simulink model "Back2BackSim1"  (R2017a)
settings: Solver=VariableStepAuto  StartTime=0.0  StopTime=.2  RelTol=1e-3
undefined symbols (not defined in the file or in its folder): st_time3
libraries: fl_lib x62, nesl_utility x32, powerlib_meascontrol x8, powerlib x1, elec_lib x1
(part 2 of 2)

== matlab function Back2BackSim1/PowerControlLoop_4CSI/Instantaneous p-q transformation ==
  data: va input; p output; vb input; vc input; ia input; ib input; ic input; q output; p0 output; iac output; ibc output; icc output; ialphC output; ibetaC output; ValA output; VbetA output
function [p, q, p0, iac, ibc, icc, ialphC, ibetaC, ValA, VbetA] = fcn(va, vb, vc, ia, ib, ic)
% Esta funcion calcula la potencia activa y reactiva instantanea
% dados 3 tensiones y 3 corrientes instantaneas.
% para esto se usa version de la transformada de clarke cuya potencia es 
% invariante (power invariant clarke transform).


pi_clarke = [[1 -1/2 -1/2]; [0 sqrt(3)/2 -sqrt(3)/2]; [1/sqrt(2) 1/sqrt(2) 1/sqrt(2)]]*sqrt(2/3);%matriz de clarke

tv = pi_clarke*[va;vb;vc];% transformada de las tensiones
ti = pi_clarke*[ia;ib;ic];%trasnformada de las corrientes

valph = tv(1);% se separa los valores de las transformadas de tension
vbet = tv(2);
v0 = tv(3);

ValA = valph;
VbetA = vbet;

ialph = ti(1);% se separa los valores de la transformda de corriente
ibet = ti(2);
i0 = ti(3);

paux=valph*ialph+vbet*ibet;
if(paux > 20e4)
    paux=20e4;
end;
if(paux < -20e4)
    paux = -20e-4;
end;

p = paux; % potencia activa instantanea

qaux=vbet*ialph-valph*ibet;

if(qaux>20e4)
    qaux=20e4;
end;
if(qaux<-20e4)
    qaux=-20e4;
end;
q = qaux; % potencia reactiva instantanea


p0 = v0*i0; % potencia instantanea de secuencia 0.



mat2cur = [valph vbet; vbet valph]; % matriz para pasar de potencia
% a corrientes por medio de una matriz de tensiones en alpha beta.

det = 1/(valph^2+vbet^2); % constante auxiliar
if(abs(det)<=100*eps(0))
    det=10*eps(0);
end;

mat2cur = mat2cur*det; % matriz final para pasar a corrientes



IabetC = mat2cur*[0; -q]; % vector corriente de compensacion en alpha beta

%inv_clarke = inv([[1 -1/2 -1/2]; [0 sqrt(3)/2 -sqrt(3)/2]; [1/sqrt(2) 1/sqrt(2) 1/sqrt(2)]]*sqrt(2/3));%matriz de clarke

ialphCaux = IabetC(1);
ibetaCaux = IabetC(2);

ilim=10e3;

if(ialphCaux>ilim)
    ialphCaux=ilim;
end;
if(ialphCaux<-ilim)
    ialphCaux =-ilim;    
end;
if(isnan(ialphCaux))
    ialphCaux=0;
end;
%---------------------
if(ibetaCaux>ilim)
    ibetaCaux=ilim;
end;
if(ibetaCaux<-ilim)
    ibetaCaux=-ilim;    
end;
if(isnan(ibetaCaux))
    ibetaCaux=0;
end;
ialphC = ialphCaux;
ibetaC = ibetaCaux;


Icom = pi_clarke\[IabetC(1); IabetC(2); 0];

iacaux = Icom(1);
ibcaux = Icom(2);
iccaux = Icom(3);

if(iacaux>ilim)
    iacaux=ilim;
end;
if(iacaux<-ilim)
    iacaux =-ilim;    
end;
if(isnan(iacaux))
    iacaux=0;
end;
%---------------------
if(ibcaux>ilim)
    ibcaux=ilim;
end;
if(ibcaux<-ilim)
    ibcaux =-ilim;    
end;

if(isnan(ibcaux))
    ibcaux=0;
end;
%-------------
if(iccaux>ilim)
    iccaux=ilim;
end;
if(iccaux<-ilim)
    iccaux =-ilim;    
end;

if(isnan(iccaux))
    iccaux=0;
end;
%-----------------
iac = iacaux;
ibc = ibcaux;
icc = iccaux;

== matlab function Back2BackSim1/PowerControlLoop_4CSI/PQ2AlphBetaCurrents ==
  data: Va input; Ia output; Vb input; p input; q input; Ib output
function [Ia, Ib] = fcn(Va, Vb, p, q)
%#codegen

% divide by zero protection
if(abs((Va^2+Vb^2))<=1000*eps(0))
    det = 1/eps(0);
else
    det = 1/(Va^2+Vb^2); % constante auxiliar
end;
%det = 1/(Va^2+Vb^2);

Mat = det*[Va Vb; Vb -Va];
Iab = Mat*[p;q];

Iaaux = Iab(1);
Ibaux = Iab(2);

ilim=1e3;

if(Iaaux>ilim)
    Iaaux=ilim;
end;
if(Iaaux<-ilim)
    Iaaux =-ilim;    
end;

if(isnan(Iaaux))
    Iaaux=0;
end;
%-----------------


if(Ibaux>ilim)
    Ibaux=ilim;
end;
if(Ibaux<-ilim)
    Ibaux =-ilim;    
end;

if(isnan(Ibaux))
    Ibaux=0;
end;
%-----------------


Ia = Iaaux;
Ib = Ibaux;
